simulink subsystem "Trajectory"  (R2024a)
settings: Solver=VariableStepAuto  StartTime=0.0  StopTime=10.0  RelTol=1e-3
undefined symbols (not defined in the file): DiscIntNeverNeededParam, MPC
libraries: ros2lib x5, robotcorelib x2, simulink x1
settings Model: Creator=Lamarre  LastModifiedBy=root
settings SolverCC: AlgebraicLoopSolver=TrustRegion
settings DebuggingCC: UnconnectedInputMsg=warning  UnconnectedOutputMsg=warning  UnconnectedLineMsg=warning
settings ModelReferenceCC: EnableRefExpFcnMdlSchedulingChecks=on
settings RTWCC: GPUComputeCapability=3.5  DLArmComputeVersion=19.05

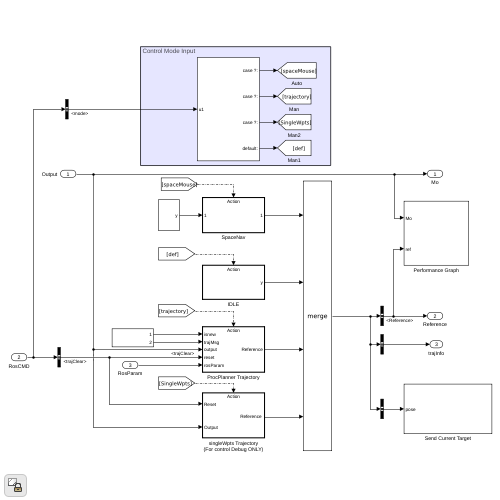
[thumbnail: Simulink's stored preview of the top-level diagram]
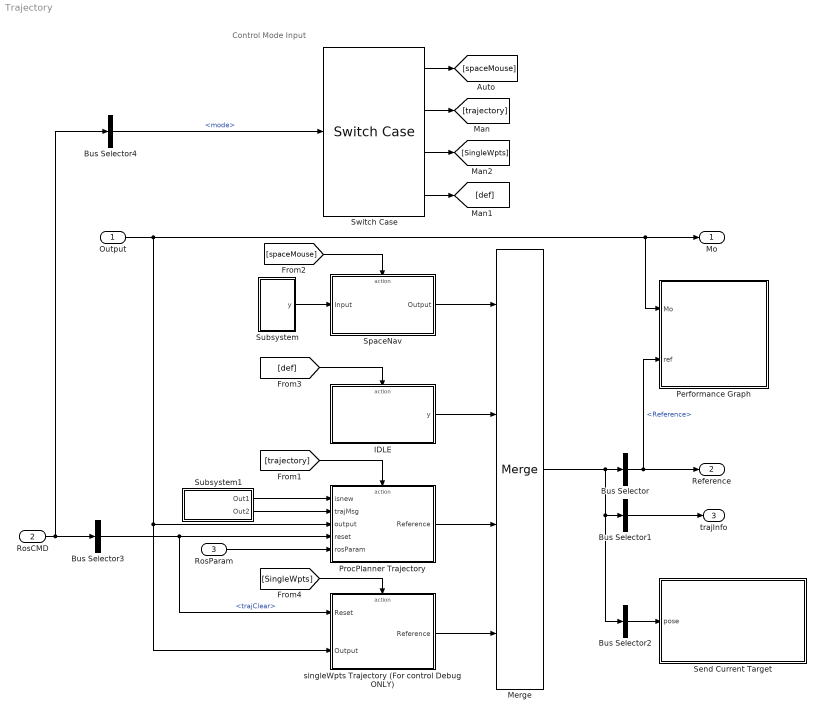
== system Trajectory ==
  note: Control Mode Input
  Output : Inport
  RosCMD : Inport  Port=2
  RosParam : Inport  Port=3
  Bus Selector : BusSelector  OutputSignals=Reference
  Bus Selector1 : BusSelector  OutputSignals=isReached,isTrajDone  OutputAsBus=on
  Bus Selector2 : BusSelector  OutputSignals=target  OutputAsBus=on
  Bus Selector3 : BusSelector  OutputSignals=trajClear
  Bus Selector4 : BusSelector  OutputSignals=mode
  IDLE : Subsystem  TreatAsAtomicUnit=on
  Merge : Merge  Inputs=4
  Performance Graph : Subsystem
  ProcPlanner Trajectory : Subsystem
  Send Current Target : Subsystem
  SpaceNav : Subsystem
  Subsystem : Subsystem
  Subsystem1 : Subsystem
  Switch Case : SwitchCase  CaseConditions={mode.traj.SpaceMouseMode,mode.traj.trajMode, mode.traj.singleWpts,}
  singleWpts Trajectory (For control Debug ONLY) : Subsystem
  Mo : Outport
  Reference : Outport  Port=2
  trajInfo : Outport  Port=3
  wires:
  Output/1 -> singleWpts Trajectory (For control Debug ONLY)/2(Output), ProcPlanner Trajectory/3(output), Mo/1, Performance Graph/1(Mo)
  Bus Selector4/1 -> Switch Case/1  "<mode>"
  [trajectory] -> ProcPlanner Trajectory/Action
  SpaceNav/1(Output) -> Merge/1
  Subsystem/1(y) -> SpaceNav/1(Input)
  [spaceMouse] -> SpaceNav/Action
  Switch Case/1 -> [spaceMouse]
  Switch Case/2 -> [trajectory]
  [def] -> IDLE/Action
  IDLE/1(y) -> Merge/2
  Switch Case/4 -> [def]
  Switch Case/3 -> [SingleWpts]
  [SingleWpts] -> singleWpts Trajectory (For control Debug ONLY)/Action
  singleWpts Trajectory (For control Debug ONLY)/1("Reference ") -> Merge/4
  ProcPlanner Trajectory/1(Reference) -> Merge/3
  Subsystem1/1(Out1) -> ProcPlanner Trajectory/1(isnew)
  Subsystem1/2(Out2) -> ProcPlanner Trajectory/2(trajMsg)
  Merge/1 -> Bus Selector/1, Bus Selector1/1, Bus Selector2/1
  Bus Selector/1 -> Reference/1, Performance Graph/2(ref)  "<Reference>"
  Bus Selector1/1 -> trajInfo/1
  Bus Selector2/1 -> Send Current Target/1(pose)
  Bus Selector3/1 -> ProcPlanner Trajectory/4(reset), singleWpts Trajectory (For control Debug ONLY)/1(Reset)  "<trajClear>"
  RosCMD/1 -> Bus Selector3/1, Bus Selector4/1
  RosParam/1 -> ProcPlanner Trajectory/5(rosParam)

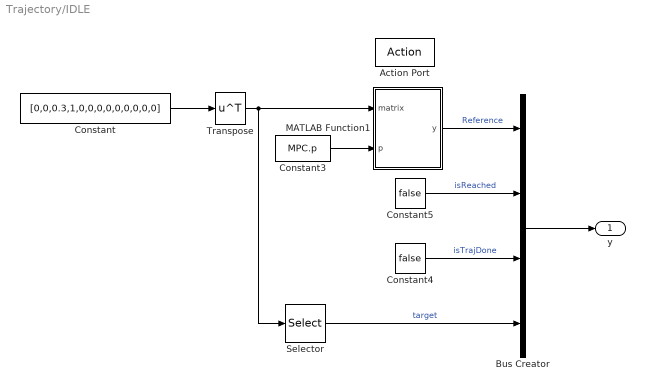
== system Trajectory/IDLE ==
  Action Port : ActionPort
  Bus Creator : BusCreator  Inputs=4
  Constant : Constant  Value=[0,0,0.3,1,0,0,0,0,0,0,0,0,0]
  Constant3 : Constant  Value=MPC.p
  Constant4 : Constant  Value=false  OutDataTypeStr=boolean
  Constant5 : Constant  Value=false  OutDataTypeStr=boolean
  MATLAB Function1 : MATLAB Function  TreatAsAtomicUnit=on
  Selector : Selector  InputPortWidth=13  IndexOptions=Index vector (dialog)  Indices=[1:7]  OutputSizes=1
  Transpose : Math  Operator=transpose
  y : Outport
  wires:
  Selector/1 -> Bus Creator/4  "target"
  Transpose/1 -> MATLAB Function1/1(matrix), Selector/1
  Constant4/1 -> Bus Creator/3  "isTrajDone"
  Constant5/1 -> Bus Creator/2  "isReached"
  Bus Creator/1 -> y/1
  MATLAB Function1/1(y) -> Bus Creator/1  "Reference"
  Constant3/1 -> MATLAB Function1/2(p)
  Constant/1 -> Transpose/1

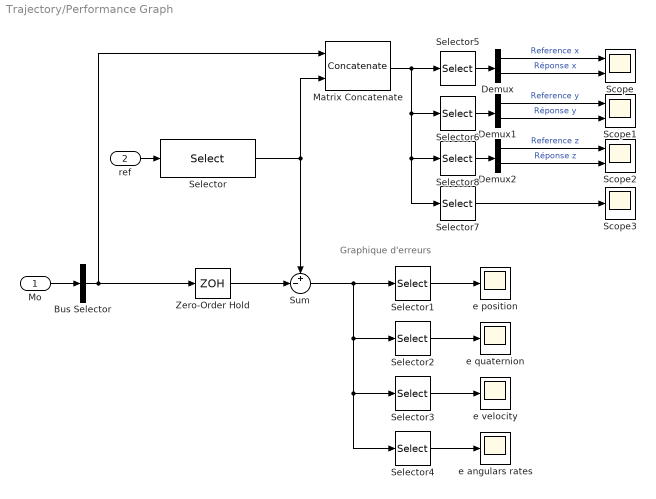
== system Trajectory/Performance Graph ==
  note: Graphique d'erreurs
  Mo : Inport
  ref : Inport  Port=2
  Bus Selector : BusSelector  OutputSignals=WorldPosition,qS2W,Body Velocity,Angular Rate  OutputAsBus=on
  Demux : Demux  Outputs=2
  Demux1 : Demux  Outputs=2
  Demux2 : Demux  Outputs=2
  Matrix Concatenate : Concatenate  Mode=Multidimensional array
  Scope : Scope  NumInputPorts=2
  Scope1 : Scope  NumInputPorts=2
  Scope2 : Scope  NumInputPorts=2
  Scope3 : Scope
  Selector : Selector  NumberOfDimensions=2  InputPortWidth=3  IndexOptions=Index vector (dialog),Index vector (dialog)  Indices=1,[1 : 13]  OutputSizes=1,1
  Selector1 : Selector  InputPortWidth=13  IndexOptions=Index vector (dialog)  Indices=[1:3]  OutputSizes=1
  Selector2 : Selector  InputPortWidth=13  IndexOptions=Index vector (dialog)  Indices=[4:7]  OutputSizes=1
  Selector3 : Selector  InputPortWidth=13  IndexOptions=Index vector (dialog)  Indices=[8:10]  OutputSizes=1
  Selector4 : Selector  InputPortWidth=13  IndexOptions=Index vector (dialog)  Indices=[10:13]  OutputSizes=1
  Selector5 : Selector  NumberOfDimensions=2  InputPortWidth=13  IndexOptions=Index vector (dialog),Index vector (dialog)  Indices=[1:2],1  OutputSizes=1,1
  Selector6 : Selector  NumberOfDimensions=2  InputPortWidth=13  IndexOptions=Index vector (dialog),Index vector (dialog)  Indices=[1:2],2  OutputSizes=1,1
  Selector7 : Selector  NumberOfDimensions=2  InputPortWidth=13  IndexOptions=Index vector (dialog),Index vector (dialog)  Indices=[1:2],[4:7]  OutputSizes=1,1
  Selector8 : Selector  NumberOfDimensions=2  InputPortWidth=13  IndexOptions=Index vector (dialog),Index vector (dialog)  Indices=[1:2],3  OutputSizes=1,1
  Sum : Sum  Inputs=+-|
  Zero-Order Hold : ZeroOrderHold  SampleTime=MPC.Ts
  e angulars rates : Scope
  e position : Scope
  e quaternion : Scope
  e velocity : Scope
  wires:
  Selector7/1 -> Scope3/1
  Zero-Order Hold/1 -> Sum/2
  Matrix Concatenate/1 -> Selector5/1, Selector6/1, Selector8/1, Selector7/1
  Demux2/2 -> Scope2/2  "Réponse z"
  Selector8/1 -> Demux2/1
  Demux2/1 -> Scope2/1  "Reference z"
  Selector6/1 -> Demux1/1
  Demux1/1 -> Scope1/1  "Reference y"
  Demux1/2 -> Scope1/2  "Réponse y"
  Demux/2 -> Scope/2  "Réponse x"
  Demux/1 -> Scope/1  "Reference x"
  Selector5/1 -> Demux/1
  Bus Selector/1 -> Zero-Order Hold/1, Matrix Concatenate/1
  Selector4/1 -> e angulars rates/1
  Selector3/1 -> e velocity/1
  Selector2/1 -> e quaternion/1
  Selector1/1 -> e position/1
  Sum/1 -> Selector1/1, Selector2/1, Selector4/1, Selector3/1
  Mo/1 -> Bus Selector/1
  Selector/1 -> Matrix Concatenate/2, Sum/1
  ref/1 -> Selector/1

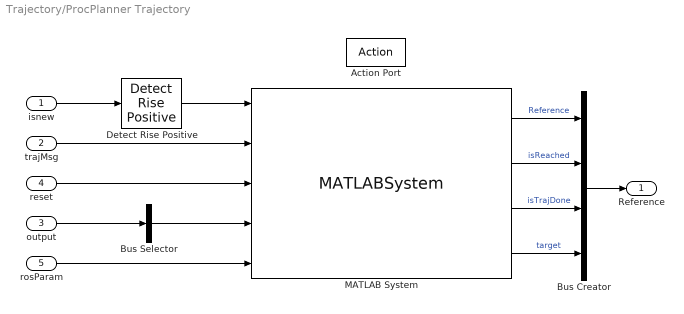
== system Trajectory/ProcPlanner Trajectory ==
  isnew : Inport
  trajMsg : Inport  Port=2
  output : Inport  Port=3
  reset : Inport  Port=4
  rosParam : Inport  Port=5
  Action Port : ActionPort
  Bus Creator : BusCreator  Inputs=4
  Bus Selector : BusSelector  OutputSignals=WorldPosition,qS2W,Body Velocity,Angular Rate  OutputAsBus=on
  Detect Rise Positive : simulink/Logic and Bit Operations/Detect Rise Positive  vinit=0  OutDataTypeStr=boolean
  MATLAB System : MATLABSystem  System=ProcPlannerManager  mpcConst=MPC  SimulateUsing=Code generation
      mask Type: ProcPlannerManager
      mask Display:
      | disp('ProcPlannerManager');
      | port_label('input',1,'isNew');
      | port_label('input',2,'trajMsg');
      | port_label('input',3,'reset');
      | port_label('input',4,'mesuredPose');
      | port_label('input',5,'mpcParams');
      | port_label('output',1,'currentPose');
      | port_label('output',2,'isReached');
      | port_label('output',3,'isTrajDone');
      | port_label('output',4,'initWpt');
  Reference : Outport
  wires:
  rosParam/1 -> MATLAB System/5
  Bus Creator/1 -> Reference/1
  MATLAB System/3 -> Bus Creator/3  "isTrajDone"
  MATLAB System/1 -> Bus Creator/1  "Reference"
  MATLAB System/2 -> Bus Creator/2  "isReached"
  trajMsg/1 -> MATLAB System/2
  Detect Rise Positive/1 -> MATLAB System/1
  MATLAB System/4 -> Bus Creator/4  "target"
  Bus Selector/1 -> MATLAB System/4
  output/1 -> Bus Selector/1
  isnew/1 -> Detect Rise Positive/1
  reset/1 -> MATLAB System/3

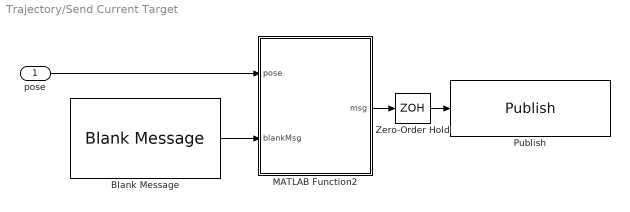
== system Trajectory/Send Current Target ==
  pose : Inport
  Blank Message : ros2lib/Blank Message  messageClass=Message  entityType=geometry_msgs/Pose  messageType=geometry_msgs/Pose  SampleTime=inf
  MATLAB Function2 : MATLAB Function  TreatAsAtomicUnit=on  SystemSampleTime=MPC.Ts
  Publish : ros2lib/Publish  topicSource=Specify your own  topic=/proc_control/current_target  messageType=geometry_msgs/Pose  QOSHistory=Keep last  QOSDepth=1  QOSReliability=Reliable  QOSDurability=Volatile  QOSDeadline=Inf  QOSLifespan=Inf  QOSLiveliness=Automatic  QOSLeaseDuration=Inf  QOSAvoidROSNamespaceConventions=off
  Zero-Order Hold : ZeroOrderHold
  wires:
  MATLAB Function2/1(msg) -> Zero-Order Hold/1
  Blank Message/1 -> MATLAB Function2/2(blankMsg)
  Zero-Order Hold/1 -> Publish/1
  pose/1 -> MATLAB Function2/1(pose)

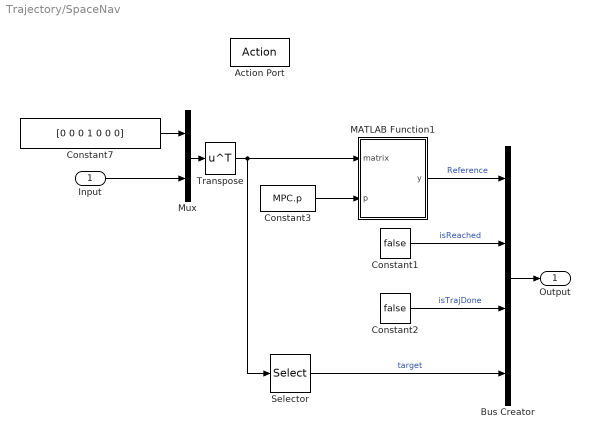
== system Trajectory/SpaceNav ==
  Input : Inport
  Action Port : ActionPort
  Bus Creator : BusCreator  Inputs=4
  Constant1 : Constant  Value=false  OutDataTypeStr=boolean
  Constant2 : Constant  Value=false  OutDataTypeStr=boolean
  Constant3 : Constant  Value=MPC.p
  Constant7 : Constant  Value=[0 0 0 1 0 0 0]
  MATLAB Function1 : MATLAB Function  TreatAsAtomicUnit=on
  Mux : Mux  Inputs=2
  Selector : Selector  InputPortWidth=13  IndexOptions=Index vector (dialog)  Indices=[1:7]  OutputSizes=1
  Transpose : Math  Operator=transpose  OutputSignalType=real
  Output : Outport
  wires:
  Selector/1 -> Bus Creator/4  "target"
  Transpose/1 -> MATLAB Function1/1(matrix), Selector/1
  Bus Creator/1 -> Output/1
  MATLAB Function1/1(y) -> Bus Creator/1  "Reference"
  Constant1/1 -> Bus Creator/2  "isReached"
  Constant2/1 -> Bus Creator/3  "isTrajDone"
  Mux/1 -> Transpose/1
  Constant3/1 -> MATLAB Function1/2(p)
  Input/1 -> Mux/2
  Constant7/1 -> Mux/1

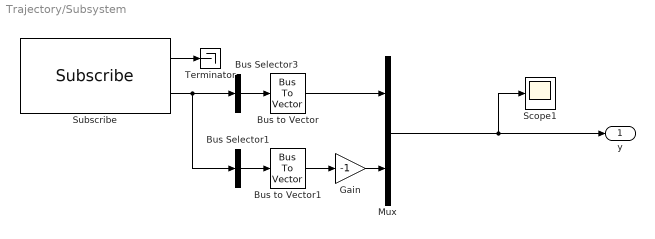
== system Trajectory/Subsystem ==
  Bus Selector1 : BusSelector  OutputSignals=Angular.X,Angular.Y,Angular.Z  OutputAsBus=on
  Bus Selector3 : BusSelector  OutputSignals=Linear.X,Linear.Y,Linear.Z  OutputAsBus=on
  Bus to Vector : BusToVector
  Bus to Vector1 : BusToVector
  Gain : Gain  Gain=-1
  Mux : Mux  Inputs=2
  Scope1 : Scope
  Subscribe : ros2lib/Subscribe  topicSource=Specify your own  topic=/spacenav/twist  messageType=geometry_msgs/Twist  sampleTime=1/25  QOSHistory=Keep last  QOSDepth=1  QOSReliability=Reliable  QOSDurability=Volatile  QOSDeadline=Inf  QOSLifespan=Inf  QOSLiveliness=Automatic  QOSLeaseDuration=Inf  QOSAvoidROSNamespaceConventions=off
  Terminator : Terminator
  y : Outport
  wires:
  Bus to Vector/1 -> Mux/1
  Gain/1 -> Mux/2
  Bus to Vector1/1 -> Gain/1
  Bus Selector1/1 -> Bus to Vector1/1
  Bus Selector3/1 -> Bus to Vector/1
  Subscribe/1 -> Terminator/1
  Subscribe/2 -> Bus Selector3/1, Bus Selector1/1
  Mux/1 -> Scope1/1, y/1

== system Trajectory/Subsystem1 ==
  Subscribe1 : ros2lib/Subscribe  topicSource=Specify your own  topic=/proc_planner/send_trajectory_list  messageType=geometry_msgs/Point  sampleTime=2  QOSHistory=Keep last  QOSDepth=1  QOSReliability=Reliable  QOSDurability=Volatile  QOSDeadline=Inf  QOSLifespan=Inf  QOSLiveliness=Automatic  QOSLeaseDuration=Inf  QOSAvoidROSNamespaceConventions=off
  Out1 : Outport
  Out2 : Outport  Port=2
  wires:
  Subscribe1/2 -> Out2/1
  Subscribe1/1 -> Out1/1

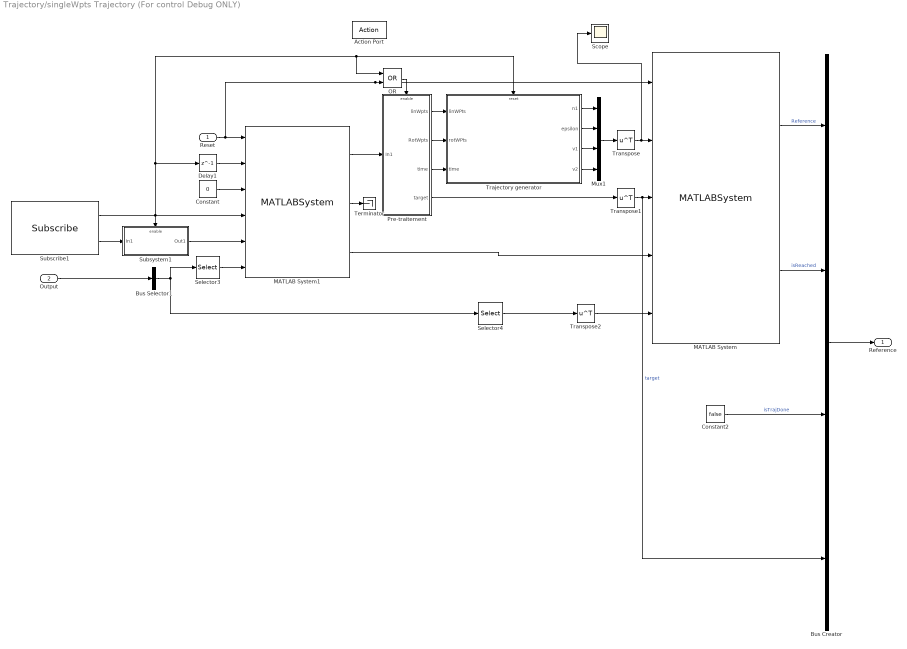
== system Trajectory/singleWpts Trajectory (For control Debug ONLY) ==
  Reset : Inport
  Output : Inport  Port=2
  Action Port : ActionPort  InitializeStates=reset
  Bus Creator : BusCreator  Inputs=4
  Bus Selector1 : BusSelector  OutputSignals=WorldPosition,qS2W,Body Velocity,Angular Rate  OutputAsBus=on
  Constant : Constant  Value=0
  Constant2 : Constant  Value=false  OutDataTypeStr=boolean
  Delay1 : Delay  DelayLength=1
  MATLAB System : MATLABSystem  System=TrajectoryManager  SampleTime=MPC.Ts  OffsetTime=0  prediction=MPC.p  bufferSize=6001  linearConvergence=.25  quaternionConvergence=.22  TargetThreshold=2  SimulateUsing=Code generation
      mask Type: TrajectoryManager
      mask Display:
      | disp('TrajectoryManager');
      | port_label('input',1,'reset');
      | port_label('input',2,'poses');
      | port_label('input',3,'target');
      | port_label('input',4,'x0');
      | port_label('input',5,'mesuredPose');
      | port_label('output',1,'currentPose');
      | port_label('output',2,'isReached');
  MATLAB System1 : MATLABSystem  System=AddPose  buffSize=2  elementSize=9  SimulateUsing=Code generation
      mask Type: AddPose
      mask Display:
      | disp('AddPose');
      | port_label('input',1,'reset');
      | port_label('input',2,'compute');
      | port_label('input',3,'clearBuffer');
      | port_label('input',4,'isNew');
      | port_label('input',5,'waypoint');
      | port_label('input',6,'xk');
      | port_label('output',1,'waypoints');
      | port_label('output',2,'count');
      | port_label('output',3,'initCond');
  Mux1 : Mux
  OR : Logic  Operator=OR  AllPortsSameDT=off  OutDataTypeStr=boolean
  Pre-traitement : Subsystem
  Scope : Scope
  Selector3 : Selector  InputPortWidth=13  IndexOptions=Index vector (dialog)  Indices=[1:7]  OutputSizes=1
  Selector4 : Selector  InputPortWidth=13  IndexOptions=Index vector (dialog)  Indices=[1:13]  OutputSizes=1
  Subscribe1 : ros2lib/Subscribe  topicSource=Specify your own  topic=/proc_control/add_pose  messageType=sonia_common_ros2/Pose  sampleTime=-1  QOSHistory=Keep last  QOSDepth=1  QOSReliability=Reliable  QOSDurability=Volatile  QOSDeadline=Inf  QOSLifespan=Inf  QOSLiveliness=Automatic  QOSLeaseDuration=Inf  QOSAvoidROSNamespaceConventions=off
  Subsystem1 : Subsystem
  Terminator : Terminator
  Trajectory generator : Subsystem
  Transpose : Math  Operator=transpose
  Transpose1 : Math  Operator=transpose
  Transpose2 : Math  Operator=transpose
  "Reference " : Outport
  wires:
  Constant2/1 -> Bus Creator/3  "isTrajDone"
  MATLAB System1/2 -> Terminator/1
  Reset/1 -> MATLAB System1/1, OR/2, MATLAB System/1
  Selector3/1 -> MATLAB System1/6
  Subsystem1/1(Out1) -> MATLAB System1/5
  Constant/1 -> MATLAB System1/3
  Delay1/1 -> MATLAB System1/2
  MATLAB System1/3 -> MATLAB System/4
  Transpose1/1 -> MATLAB System/3, Bus Creator/4  "target"
  Transpose/1 -> MATLAB System/2, Scope/1
  Bus Creator/1 -> "Reference "/1
  MATLAB System/1 -> Bus Creator/1  "Reference"
  Trajectory generator/1(n1) -> Mux1/1
  Trajectory generator/2(epsilon) -> Mux1/2
  Transpose2/1 -> MATLAB System/5
  Pre-traitement/4(target) -> Transpose1/1
  Trajectory generator/4(v2) -> Mux1/4
  Trajectory generator/3(v1) -> Mux1/3
  Selector4/1 -> Transpose2/1
  Mux1/1 -> Transpose/1
  Bus Selector1/1 -> Selector3/1, Selector4/1
  MATLAB System/2 -> Bus Creator/2  "isReached"
  MATLAB System1/1 -> Pre-traitement/1(In1)
  Output/1 -> Bus Selector1/1
  OR/1 -> Pre-traitement/Enable
  Pre-traitement/3(time) -> Trajectory generator/3(time)
  Pre-traitement/2(RotWpts) -> Trajectory generator/2(rotWPts)
  Pre-traitement/1(linWpts) -> Trajectory generator/1(linWPts)
  Subscribe1/1 -> MATLAB System1/4, Subsystem1/Enable, Delay1/1, OR/1, Trajectory generator/Reset
  Subscribe1/2 -> Subsystem1/1(In1)

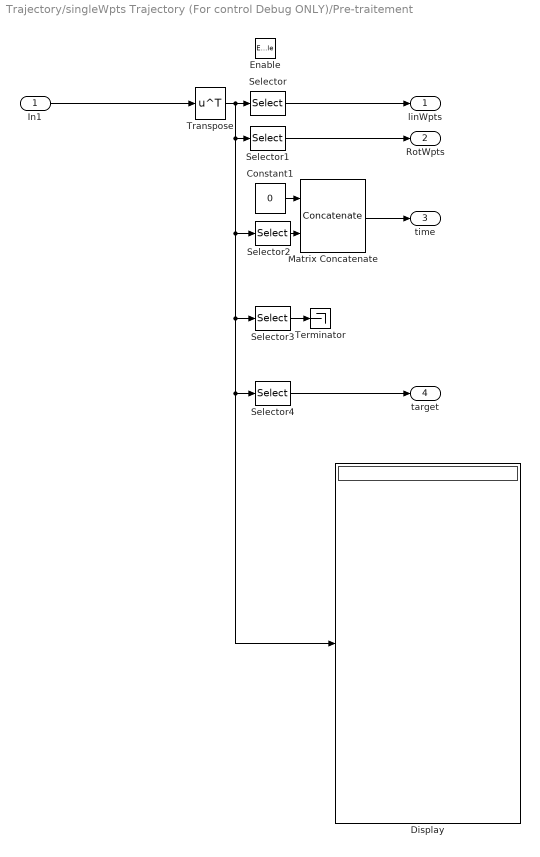
== system Trajectory/singleWpts Trajectory (For control Debug ONLY)/Pre-traitement ==
  In1 : Inport
  Enable : EnablePort
  Constant1 : Constant  Value=0
  Display : Display
  Matrix Concatenate : Concatenate  Mode=Multidimensional array
  Selector : Selector  NumberOfDimensions=2  InputPortWidth=3  IndexOptions=Index vector (dialog),Index vector (dialog)  Indices=[1:3],[1:2]  OutputSizes=1,1
  Selector1 : Selector  NumberOfDimensions=2  InputPortWidth=3  IndexOptions=Index vector (dialog),Index vector (dialog)  Indices=[4:7],[1:2]  OutputSizes=1,1
  Selector2 : Selector  NumberOfDimensions=2  InputPortWidth=3  IndexOptions=Index vector (dialog),Index vector (dialog)  Indices=[8],[2]  OutputSizes=1,1
  Selector3 : Selector  NumberOfDimensions=2  InputPortWidth=3  IndexOptions=Index vector (dialog),Index vector (dialog)  Indices=[9],[2]  OutputSizes=1,1
  Selector4 : Selector  NumberOfDimensions=2  InputPortWidth=3  IndexOptions=Index vector (dialog),Index vector (dialog)  Indices=[1:7],[2]  OutputSizes=1,1
  Terminator : Terminator
  Transpose : Math  Operator=transpose
  linWpts : Outport
  RotWpts : Outport  Port=2
  time : Outport  Port=3
  target : Outport  Port=4
  wires:
  Selector3/1 -> Terminator/1
  Selector4/1 -> target/1
  Selector1/1 -> RotWpts/1
  Matrix Concatenate/1 -> time/1
  Constant1/1 -> Matrix Concatenate/1
  Selector2/1 -> Matrix Concatenate/2
  In1/1 -> Transpose/1
  Transpose/1 -> Selector/1, Selector1/1, Display/1, Selector4/1, Selector3/1, Selector2/1
  Selector/1 -> linWpts/1

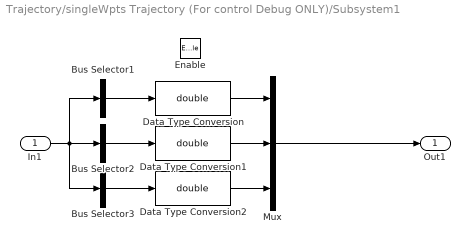
== system Trajectory/singleWpts Trajectory (For control Debug ONLY)/Subsystem1 ==
  In1 : Inport
  Enable : EnablePort
  Bus Selector1 : BusSelector  OutputSignals=Position.X,Position.Y,Position.Z,Orientation.Z,Orientation.Y,Orientation.X  OutputAsBus=on
  Bus Selector2 : BusSelector  OutputSignals=Frame,Speed  OutputAsBus=on
  Bus Selector3 : BusSelector  OutputSignals=Fine  OutputAsBus=on
  Data Type Conversion : DataTypeConversion  OutDataTypeStr=double  SaturateOnIntegerOverflow=off  RndMeth=Floor  LockScale=on
  Data Type Conversion1 : DataTypeConversion  OutDataTypeStr=double  SaturateOnIntegerOverflow=off  RndMeth=Floor  LockScale=on
  Data Type Conversion2 : DataTypeConversion  OutDataTypeStr=double  SaturateOnIntegerOverflow=off  RndMeth=Floor  LockScale=on
  Mux : Mux  Inputs=3
  Out1 : Outport
  wires:
  Mux/1 -> Out1/1
  Data Type Conversion2/1 -> Mux/3
  Data Type Conversion1/1 -> Mux/2
  Data Type Conversion/1 -> Mux/1
  Bus Selector3/1 -> Data Type Conversion2/1
  Bus Selector2/1 -> Data Type Conversion1/1
  In1/1 -> Bus Selector2/1, Bus Selector3/1, Bus Selector1/1
  Bus Selector1/1 -> Data Type Conversion/1

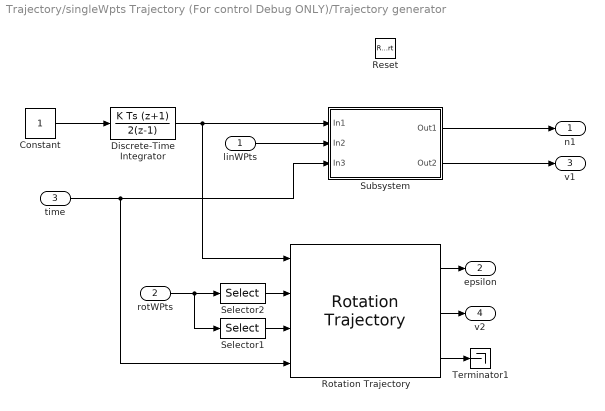
== system Trajectory/singleWpts Trajectory (For control Debug ONLY)/Trajectory generator ==
  linWPts : Inport
  rotWPts : Inport  Port=2
  time : Inport  Port=3
  Reset : ResetPort  DisableCoverage=on
  Constant : Constant
  Discrete-Time Integrator : DiscreteIntegrator  IntegratorMethod=Integration: Trapezoidal  SampleTime=-1  ICPrevOutput=DiscIntNeverNeededParam  ICPrevScaledInput=DiscIntNeverNeededParam
  Rotation Trajectory : robotcorelib/Rotation Trajectory  WaypointFormat=Quaternion  WaypointSource=External  R0=[ 1, 0, 0, 0 ]'  RF=[ 0, 0, 1, 0 ]'  TimeInterval=[ 0, 1 ]  CustomTimeScaling=off  ParameterSource=Internal  TSTime=0:0.1:1  TimeScaling=[ 0:0.1:1; ones( 1, 11 ); zeros( 1, 11 ) ]  SimulateUsing=Code generation
  Selector1 : Selector  NumberOfDimensions=2  InputPortWidth=3  IndexOptions=Index vector (dialog),Index vector (dialog)  Indices=[1:4],2  OutputSizes=1,1
  Selector2 : Selector  NumberOfDimensions=2  InputPortWidth=3  IndexOptions=Index vector (dialog),Index vector (dialog)  Indices=[1:4],1  OutputSizes=1,1
  Subsystem : Subsystem
  Terminator1 : Terminator
  n1 : Outport
  epsilon : Outport  Port=2
  v1 : Outport  Port=3
  v2 : Outport  Port=4
  wires:
  Rotation Trajectory/2 -> v2/1
  Subsystem/2(Out2) -> v1/1
  Subsystem/1(Out1) -> n1/1
  Rotation Trajectory/1 -> epsilon/1
  Selector1/1 -> Rotation Trajectory/3
  Selector2/1 -> Rotation Trajectory/2
  rotWPts/1 -> Selector2/1, Selector1/1
  Rotation Trajectory/3 -> Terminator1/1
  time/1 -> Subsystem/3(In3), Rotation Trajectory/4
  linWPts/1 -> Subsystem/2(In2)
  Discrete-Time Integrator/1 -> Subsystem/1(In1), Rotation Trajectory/1
  Constant/1 -> Discrete-Time Integrator/1

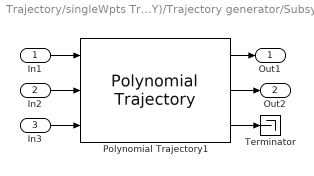
== system Trajectory/singleWpts Trajectory (For control Debug ONLY)/Trajectory generator/Subsystem ==
  In1 : Inport
  In2 : Inport  Port=2
  In3 : Inport  Port=3
  Polynomial Trajectory1 : robotcorelib/Polynomial Trajectory  WaypointSource=External  Waypoints=wayPoints  TimePoints=[ 0, 1, 2, 3, 4 ]  TimeInterval=[0,5]  Method=Cubic Polynomial  ParameterSource=Internal  VelocityBoundaryCondition=zeros( 3, 2 )  AccelerationBoundaryCondition=zeros( 2, 5 )  SimulateUsing=Code generation
  Terminator : Terminator
  Out1 : Outport
  Out2 : Outport  Port=2
  wires:
  Polynomial Trajectory1/2 -> Out2/1
  In3/1 -> Polynomial Trajectory1/3
  Polynomial Trajectory1/1 -> Out1/1
  Polynomial Trajectory1/3 -> Terminator/1
  In1/1 -> Polynomial Trajectory1/1
  In2/1 -> Polynomial Trajectory1/2

== matlab function Trajectory/Send Current Target/MATLAB Function2 ==
  data: pose input; blankMsg input; msg output Bus: SL_Bus_proc_control_geometry_msgs_Pose
function msg = assignInitialWpts(pose, blankMsg)
msg = blankMsg;
msg.Position.X = pose(1);
msg.Position.Y = pose(2);
msg.Position.Z = pose(3);

msg.Orientation.W = pose(4);
msg.Orientation.X = pose(5);
msg.Orientation.Y = pose(6);
msg.Orientation.Z = pose(7);

== matlab function Trajectory/IDLE/MATLAB Function1 ==
  data: matrix input; y output size=[10 13]; p input
function y = fcn(matrix,p)
matrix(10)=-matrix(10);
y = repmat(matrix,10,1);

== matlab function Trajectory/SpaceNav/MATLAB Function1 ==
  data: matrix input; y output size=[10 13]; p input
function y = fcn(matrix,p)
%matrix(10)=-matrix(10);
y = repmat(matrix,10,1);
